simulink model "sinal2016a"  (R2016a)
settings: Solver=VariableStepAuto  SolverMode=SingleTasking  StartTime=0.0  StopTime=0.01667*2  MaxStep=1e-4  RelTol=1e-3
libraries: fl_lib x14, nesl_utility x7, powerlib_meascontrol x3, pe_lib x2
settings Model: Creator=aluno  LastModifiedBy=Victor
settings DebuggingCC: SFUnexpectedBacktrackingDiag=error  SFNoUnconditionalDefaultTransitionDiag=error
settings GRTTargetCC: TargetLangStandard=C99 (ISO)  GeneratePreprocessorConditionals=Use local settings
settings ConfigComp: CovMetricSettings=dwe  CovHtmlReporting=off  CovSaveCumulativeToWorkspaceVar=off  CovSaveSingleToWorkspaceVar=off  CovExternalEMLEnable=on

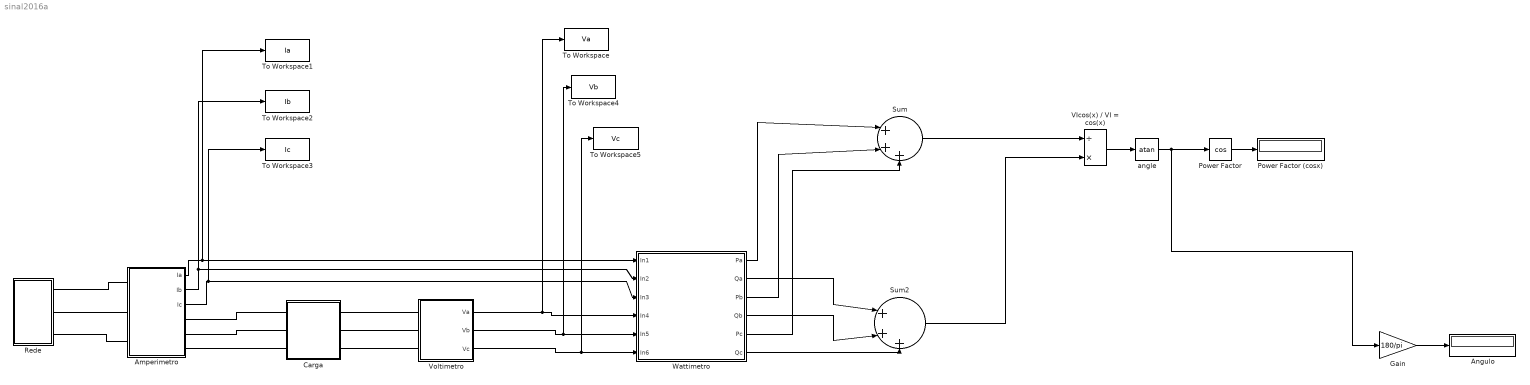
== system sinal2016a ==
  Amperimetro : Subsystem
  Angulo : Display
  Carga : Subsystem
  Gain : Gain  Gain=180/pi
  Power Factor : Trigonometry  Operator=cos  OutputSignalType=real
  Power Factor (cosx) : Display
  "Rede " : Subsystem
  Sum : Sum  Inputs=|+++
  Sum2 : Sum  Inputs=|+++
  To Workspace : ToWorkspace  VariableName=Va  SampleTime=1/18000
  To Workspace1 : ToWorkspace  VariableName=Ia  SampleTime=1/18000
  To Workspace2 : ToWorkspace  VariableName=Ib  SampleTime=1/18000
  To Workspace3 : ToWorkspace  VariableName=Ic  SampleTime=1/18000
  To Workspace4 : ToWorkspace  VariableName=Vb  SampleTime=1/18000
  To Workspace5 : ToWorkspace  VariableName=Vc  SampleTime=1/18000
  VIcos(x) / VI = cos(x) : Product  Inputs=/*
  Voltimetro : Subsystem
  Wattimetro : Subsystem
  angle : Trigonometry  Operator=atan  OutputSignalType=real
  wires:
  Gain/1 -> Angulo/1
  angle/1 -> Gain/1, Power Factor/1
  Power Factor/1 -> Power Factor (cosx)/1
  VIcos(x) / VI = cos(x)/1 -> angle/1
  Amperimetro/1(Ia) -> To Workspace1/1, Wattimetro/1(In1)
  Amperimetro/2("Ib ") -> To Workspace2/1, Wattimetro/2(In2)
  Amperimetro/3(Ic) -> To Workspace3/1, Wattimetro/3(In3)
  Voltimetro/1(Va) -> Wattimetro/4(In4), To Workspace/1
  Voltimetro/2(Vb) -> To Workspace4/1, Wattimetro/5(In5)
  Voltimetro/3(Vc) -> To Workspace5/1, Wattimetro/6(In6)
  Wattimetro/1(Pa) -> Sum/1
  Wattimetro/3(Pb) -> Sum/2
  Wattimetro/5(Pc) -> Sum/3
  Sum/1 -> VIcos(x) / VI = cos(x)/1
  Wattimetro/2(Qa) -> Sum2/1
  Wattimetro/4(Qb) -> Sum2/2
  Wattimetro/6(Qc) -> Sum2/3
  Sum2/1 -> VIcos(x) / VI = cos(x)/2
  connections:
  Carga/LConn1 -- Amperimetro/RConn1
  Amperimetro/LConn1 -- "Rede "/RConn1
  Carga/LConn2 -- Amperimetro/RConn2
  Amperimetro/LConn2 -- "Rede "/RConn2
  Amperimetro/LConn3 -- "Rede "/RConn3
  Carga/LConn3 -- Amperimetro/RConn3
  Voltimetro/LConn1 -- Carga/RConn1
  Voltimetro/LConn2 -- Carga/RConn2
  Voltimetro/LConn3 -- Carga/RConn3

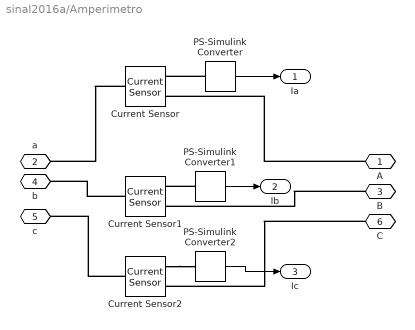
== system sinal2016a/Amperimetro ==
  Current Sensor : fl_lib/Electrical/Electrical Sensors/Current Sensor
  Current Sensor1 : fl_lib/Electrical/Electrical Sensors/Current Sensor
  Current Sensor2 : fl_lib/Electrical/Electrical Sensors/Current Sensor
  PS-Simulink Converter : nesl_utility/PS-Simulink Converter  PhysicalDomain=network_engine_domain  SubClassName=ps_output  LeftPortType=input  RightPortType=output  PseudoPeriodic=off  Frequencies=[]  Unit=A  AffineConversion=off
  PS-Simulink Converter1 : nesl_utility/PS-Simulink Converter  PhysicalDomain=network_engine_domain  SubClassName=ps_output  LeftPortType=input  RightPortType=output  PseudoPeriodic=off  Frequencies=[]  Unit=A  AffineConversion=off
  PS-Simulink Converter2 : nesl_utility/PS-Simulink Converter  PhysicalDomain=network_engine_domain  SubClassName=ps_output  LeftPortType=input  RightPortType=output  PseudoPeriodic=off  Frequencies=[]  Unit=A  AffineConversion=off
  "A " : PMIOPort  Port=1  Side=Right
  a : PMIOPort  Port=2  Side=Left
  B : PMIOPort  Port=3  Side=Right
  b : PMIOPort  Port=4  Side=Left
  c : PMIOPort  Port=5  Side=Left
  C : PMIOPort  Port=6  Side=Right
  Ia : Outport
  "Ib " : Outport  Port=2
  Ic : Outport  Port=3
  wires:
  PS-Simulink Converter/1 -> Ia/1
  PS-Simulink Converter1/1 -> "Ib "/1
  PS-Simulink Converter2/1 -> Ic/1
  connections:
  Current Sensor2/LConn1 -- c/RConn1
  Current Sensor/LConn1 -- a/RConn1
  Current Sensor2/RConn1 -- PS-Simulink Converter2/LConn1
  PS-Simulink Converter1/LConn1 -- Current Sensor1/RConn1
  Current Sensor1/LConn1 -- b/RConn1
  B/RConn1 -- Current Sensor1/RConn2
  "A "/RConn1 -- Current Sensor/RConn2
  C/RConn1 -- Current Sensor2/RConn2
  PS-Simulink Converter/LConn1 -- Current Sensor/RConn1

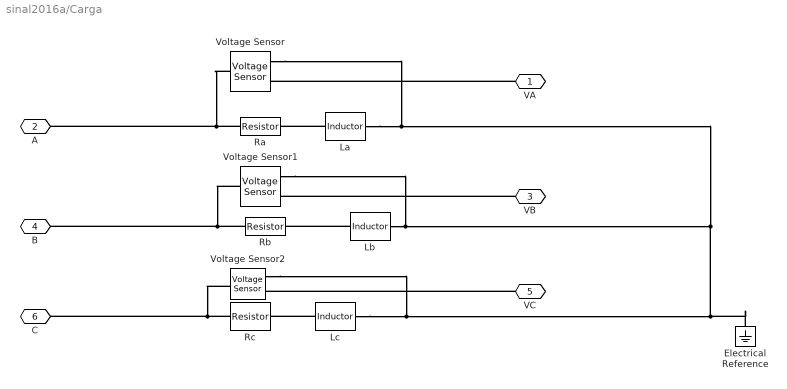
== system sinal2016a/Carga ==
  Electrical Reference : fl_lib/Electrical/Electrical Elements/Electrical Reference
  La : fl_lib/Electrical/Electrical Elements/Inductor  l=10 mH  r=0 Ohm  g=1e-9 1/Ohm  i_specify=off  i_priority=None  i=0 A  i_nominal_specify=off  i_nominal_unit=A  i_nominal_value=1  v_specify=off  v_priority=None  v=0 V  v_nominal_specify=off  v_nominal_unit=V  v_nominal_value=1  i_L_specify=off  i_L_priority=High  i_L=0 A  i_L_nominal_specify=off  i_L_nominal_unit=A  i_L_nominal_value=1
  Lb : fl_lib/Electrical/Electrical Elements/Inductor  l=10 mH  r=0 Ohm  g=1e-9 1/Ohm  i_specify=off  i_priority=None  i=0 A  i_nominal_specify=off  i_nominal_unit=A  i_nominal_value=1  v_specify=off  v_priority=None  v=0 V  v_nominal_specify=off  v_nominal_unit=V  v_nominal_value=1  i_L_specify=off  i_L_priority=High  i_L=0 A  i_L_nominal_specify=off  i_L_nominal_unit=A  i_L_nominal_value=1
  Lc : fl_lib/Electrical/Electrical Elements/Inductor  l=10 mH  r=0 Ohm  g=1e-9 1/Ohm  i_specify=off  i_priority=None  i=0 A  i_nominal_specify=off  i_nominal_unit=A  i_nominal_value=1  v_specify=off  v_priority=None  v=0 V  v_nominal_specify=off  v_nominal_unit=V  v_nominal_value=1  i_L_specify=off  i_L_priority=High  i_L=0 A  i_L_nominal_specify=off  i_L_nominal_unit=A  i_L_nominal_value=1
  Ra : fl_lib/Electrical/Electrical Elements/Resistor  R=50 Ohm  i_specify=off  i_priority=None  i=21.03000386556 A  i_nominal_specify=off  i_nominal_unit=A  i_nominal_value=12.695145924886  v_specify=off  v_priority=None  v=0 V  v_nominal_specify=off  v_nominal_unit=V  v_nominal_value=1
  Rb : fl_lib/Electrical/Electrical Elements/Resistor  R=50 Ohm  i_specify=off  i_priority=None  i=0 A  i_nominal_specify=off  i_nominal_unit=A  i_nominal_value=1  v_specify=off  v_priority=None  v=0 V  v_nominal_specify=off  v_nominal_unit=V  v_nominal_value=1
  Rc : fl_lib/Electrical/Electrical Elements/Resistor  R=50 Ohm  i_specify=off  i_priority=None  i=0 A  i_nominal_specify=off  i_nominal_unit=A  i_nominal_value=1  v_specify=off  v_priority=None  v=0 V  v_nominal_specify=off  v_nominal_unit=V  v_nominal_value=1
  Voltage Sensor : fl_lib/Electrical/Electrical Sensors/Voltage Sensor
  Voltage Sensor1 : fl_lib/Electrical/Electrical Sensors/Voltage Sensor
  Voltage Sensor2 : fl_lib/Electrical/Electrical Sensors/Voltage Sensor
  VA : PMIOPort  Port=1  Side=Right
  A : PMIOPort  Port=2  Side=Left
  VB : PMIOPort  Port=3  Side=Right
  B : PMIOPort  Port=4  Side=Left
  VC : PMIOPort  Port=5  Side=Right
  C : PMIOPort  Port=6  Side=Left
  connections:
  VC/RConn1 -- Voltage Sensor2/RConn1
  Electrical Reference/LConn1 -- Lc/RConn1 -- Voltage Sensor2/RConn2 -- Lb/RConn1 -- Voltage Sensor1/RConn2 -- La/RConn1 -- Voltage Sensor/RConn2
  VB/RConn1 -- Voltage Sensor1/RConn1
  Ra/LConn1 -- Voltage Sensor/LConn1 -- A/RConn1
  Rc/LConn1 -- Voltage Sensor2/LConn1 -- C/RConn1
  Rb/LConn1 -- Voltage Sensor1/LConn1 -- B/RConn1
  VA/RConn1 -- Voltage Sensor/RConn1
  La/LConn1 -- Ra/RConn1
  Lb/LConn1 -- Rb/RConn1
  Lc/LConn1 -- Rc/RConn1

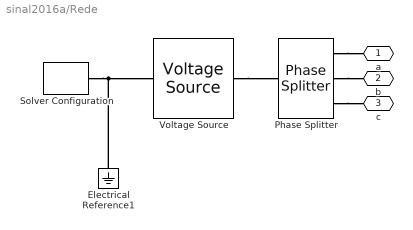
== system sinal2016a/Rede  ==
  Electrical Reference1 : fl_lib/Electrical/Electrical Elements/Electrical Reference
  Phase Splitter : pe_lib/Connections/Phase Splitter
  Solver Configuration : nesl_utility/Solver Configuration  PhysicalDomain=network_engine_domain  SubClassName=solver  LeftPortType=input  RightPortType=generic  Accelerate=off  Tones=[]  Harmonics=[]  SimulateNoise=off  Profile=off  UseLocalSampling=off  EnableSwitchedLinearOptims=on  FrequencyDomain=off  UseCCode=off  RelTol=0.001  AbsTol=1e-06  MinStep=1e-09  ToWorkspace=off  RevertToSquareIcSolve=off  NumHomotopyIterations=100  PhasorMode=off  PhasorModeNumHarmonics=1  OverrideAbsTol=off  DoDC=off  ResidualTolerance=1e-09  UseLocalSolver=on  LocalSolverChoice=NE_BACKWARD_EULER_ADVANCER  LocalSolverSampleTime=1/18000  DoFixedCost=on  MaxNonlinIter=3  MaxModeIter=2  LinearAlgebra=Sparse  DelaysMemoryBudget=1024  AutomaticFiltering=on  FilteringTimeConstant=0.001
  Voltage Source : pe_lib/Sources/Voltage Source  vline_rms=sqrt(3) * 220 / sqrt(2) V  shift=0 deg  freq=60 Hz  harmonic_option=1  harmonic_orders=[3.0, 5.0, 7.0, 9.0, 11.0, 13.0]  harmonic_ratios=[0.003, 0.01, 0.002, 0.01, 0.03, 0.01]
  a : PMIOPort  Port=1  Side=Right
  b : PMIOPort  Port=2  Side=Right
  c : PMIOPort  Port=3  Side=Right
  connections:
  Voltage Source/RConn1 -- Phase Splitter/LConn1
  Phase Splitter/RConn2 -- b/RConn1
  Phase Splitter/RConn3 -- c/RConn1
  Phase Splitter/RConn1 -- a/RConn1
  Solver Configuration/RConn1 -- Voltage Source/LConn1 -- Electrical Reference1/LConn1

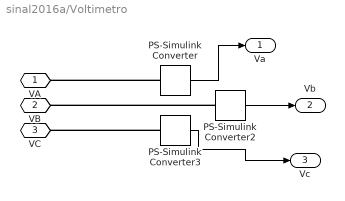
== system sinal2016a/Voltimetro ==
  PS-Simulink Converter : nesl_utility/PS-Simulink Converter  PhysicalDomain=network_engine_domain  SubClassName=ps_output  LeftPortType=input  RightPortType=output  PseudoPeriodic=off  Frequencies=[]  Unit=V  AffineConversion=off
  PS-Simulink Converter2 : nesl_utility/PS-Simulink Converter  PhysicalDomain=network_engine_domain  SubClassName=ps_output  LeftPortType=input  RightPortType=output  PseudoPeriodic=off  Frequencies=[]  Unit=V  AffineConversion=off
  PS-Simulink Converter3 : nesl_utility/PS-Simulink Converter  PhysicalDomain=network_engine_domain  SubClassName=ps_output  LeftPortType=input  RightPortType=output  PseudoPeriodic=off  Frequencies=[]  Unit=V  AffineConversion=off
  VA : PMIOPort  Port=1  Side=Left
  VB : PMIOPort  Port=2  Side=Left
  VC : PMIOPort  Port=3  Side=Left
  Va : Outport
  Vb : Outport  Port=2
  Vc : Outport  Port=3
  wires:
  PS-Simulink Converter3/1 -> Vc/1
  PS-Simulink Converter2/1 -> Vb/1
  PS-Simulink Converter/1 -> Va/1
  connections:
  PS-Simulink Converter2/LConn1 -- VB/RConn1
  PS-Simulink Converter/LConn1 -- VA/RConn1
  PS-Simulink Converter3/LConn1 -- VC/RConn1

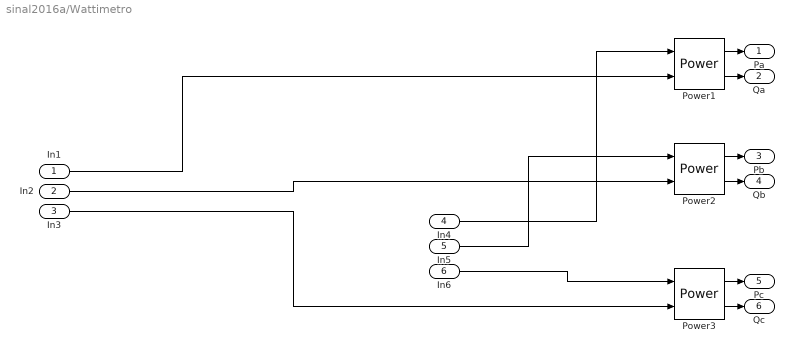
== system sinal2016a/Wattimetro ==
  In1 : Inport
  In2 : Inport  Port=2
  In3 : Inport  Port=3
  In4 : Inport  Port=4
  In5 : Inport  Port=5
  In6 : Inport  Port=6
  Power1 : powerlib_meascontrol/Measurements/Power  Freq=60  Vinit=[1, 0]  Iinit=[1, 0]  Ts=1/18000
  Power2 : powerlib_meascontrol/Measurements/Power  Freq=60  Vinit=[1, 0]  Iinit=[1, 0]  Ts=1/18000
  Power3 : powerlib_meascontrol/Measurements/Power  Freq=60  Vinit=[1, 0]  Iinit=[1, 0]  Ts=1/18000
  Pa : Outport
  Qa : Outport  Port=2
  Pb : Outport  Port=3
  Qb : Outport  Port=4
  Pc : Outport  Port=5
  Qc : Outport  Port=6
  wires:
  In4/1 -> Power1/1
  Power2/1 -> Pb/1
  Power1/2 -> Qa/1
  Power1/1 -> Pa/1
  Power3/1 -> Pc/1
  Power2/2 -> Qb/1
  Power3/2 -> Qc/1
  In6/1 -> Power3/1
  In2/1 -> Power2/2
  In1/1 -> Power1/2
  In3/1 -> Power3/2
  In5/1 -> Power2/1
